simulink model "alternateDesignSimu"  (R2015a)
settings: Solver=ode3  StartTime=0.0  StopTime=20  FixedStep=.01  RelTol=1e-3
libraries: cstblocks x6, simulink x1
settings Model: Creator=morten  LastModifiedBy=morten

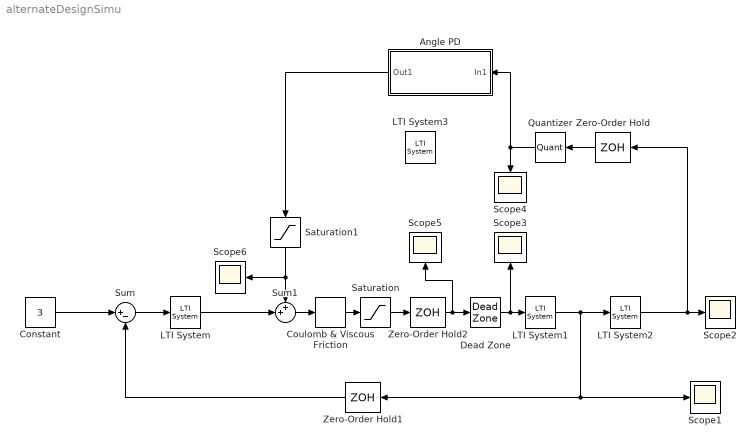
== system alternateDesignSimu ==
  Angle PD : Subsystem
  Constant : Constant  Value=3
  Coulomb & Viscous Friction : simulink/Discontinuities/Coulomb & Viscous Friction  offset=4.5  gain=1
  Dead Zone : DeadZone  LowerValue=-4.5  UpperValue=4.5  SaturateOnIntegerOverflow=on
  LTI System : cstblocks/LTI System  sys=C1  IC=[]
  LTI System1 : cstblocks/LTI System  sys=Hx  IC=[]
  LTI System2 : cstblocks/LTI System  sys=W  IC=[]
  LTI System3 : cstblocks/LTI System  sys=dC2  IC=[]
  Quantizer : Quantizer  QuantizationInterval=.001
  Saturation : Saturate  UpperLimit=12.5  LowerLimit=-12.5
  Saturation1 : Saturate  UpperLimit=10  LowerLimit=-10
  Scope{1..6} (6 alike) : Scope
      Scope2 settings: YMin=-1  YMax=1
      Scope3 settings: SaveName=ScopeData2
      Scope4 settings: SaveName=ScopeData3
      Scope5 settings: SaveName=ScopeData4
      Scope6 settings: SaveName=ScopeData5
  Sum : Sum  Inputs=|+-
  Sum1 : Sum  Inputs=++|
  Zero-Order Hold : ZeroOrderHold  SampleTime=.01
  Zero-Order Hold1 : ZeroOrderHold  SampleTime=.01
  Zero-Order Hold2 : ZeroOrderHold  SampleTime=.01
  wires:
  Sum/1 -> LTI System/1
  LTI System/1 -> Sum1/2
  Constant/1 -> Sum/1
  Sum1/1 -> Coulomb & Viscous Friction/1
  LTI System1/1 -> LTI System2/1, Zero-Order Hold1/1, Scope1/1
  LTI System2/1 -> Zero-Order Hold/1, Scope2/1
  Coulomb & Viscous Friction/1 -> Saturation/1
  Dead Zone/1 -> Scope3/1, LTI System1/1
  Zero-Order Hold1/1 -> Sum/2
  Zero-Order Hold2/1 -> Scope5/1, Dead Zone/1
  Saturation/1 -> Zero-Order Hold2/1
  Saturation1/1 -> Sum1/1, Scope6/1
  Zero-Order Hold/1 -> Quantizer/1
  Quantizer/1 -> Angle PD/1(In1), Scope4/1
  Angle PD/1(Out1) -> Saturation1/1

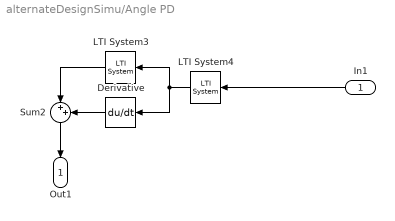
== system alternateDesignSimu/Angle PD ==
  In1 : Inport
  Derivative : Derivative
  LTI System3 : cstblocks/LTI System  sys=p  IC=[]
  LTI System4 : cstblocks/LTI System  sys=k  IC=[]
  Sum2 : Sum  Inputs=|++
  Out1 : Outport
  wires:
  Derivative/1 -> Sum2/2
  LTI System3/1 -> Sum2/1
  LTI System4/1 -> Derivative/1, LTI System3/1
  Sum2/1 -> Out1/1
  In1/1 -> LTI System4/1
